simulink model "cusCommDemo_m"  (Simulink 6.0)
settings: Solver=FixedStepDiscrete  StartTime=0.0  StopTime=48  FixedStep=1  RelTol=1e-3
PostLoadFcn:
  | INC=uint8(1);LIMIT=uint8(16);RESET=uint8(0);K=int32(2);
libraries: mptlib x1
settings Model: CovMetricSettings=d  Creator=pszpak  LastModifiedBy=lzhang  ExtModeTrigMode=oneshot  ExtModeArmWhenConnect=off  ExtModeAutoUpdateStatusClock=off  BufferReuse=off  ProdHWDeviceType=Specified
settings DataIOCC: LimitDataPoints=off  SaveFormat=StructureWithTime  SaveOutput=off  SaveTime=off  SignalLoggingName=sigsOut
settings OptimizationCC: BlockReduction=off  InlineParams=on  BufferReuse=off  EnforceIntegerDowncast=off  LifeSpan=1
settings DebuggingCC: CheckExecutionContextPreStartOutputMsg=on  CheckExecutionContextRuntimeOutputMsg=on  SignalResolutionControl=TryResolveAll  SolverPrmCheckMsg=none  IntegerOverflowMsg=none
settings HardwareCC: ProdHWDeviceType=Specified
settings ModelReferenceCC: UpdateModelReferenceTargets=IfOutOfDate
settings RTWCC: SystemTargetFile=ert.tlc  TLCOptions=-aWarnNonSaturatedBlocks=0 -p0  TemplateMakefile=ert_default_tmf  GenerateReport=on  RTWVerbose=off  ProcessScript=ert_make_rtw_hook  IncludeHyperlinkInReport=on  LaunchReport=on
settings CodeAppCC: IgnoreCustomStorageClasses=off  PrefixModelToSubsysFcnNames=off  MangleLength=5  CustomCommentsFcn=custom_comments_example.m  EnableCustomComments=on
settings ERTTargetCC: TargetFcnLib=ansi_tfl_tmw.mat  GenFloatMathFcnCalls=ANSI_C  GenerateSampleERTMain=on  IncludeMdlTerminateFcn=off  SuppressErrorStatus=on  SupportContinuousTime=on  SupportNonInlinedSFcns=on  RootIOFormat=Individual Arguments  ERTSrcFileBannerTemplate=example_banner.tlc  ERTHdrFileBannerTemplate=example_banner.tlc  ERTDataSrcFileTemplate=example_banner.tlc  ERTDataHdrFileTemplate=example_banner.tlc  ERTCustomFileTemplate=example_file_process.tlc  InitialValueSource=DataObject
settings SFSimCC: SFSimApplyToAllLibs=on  SFSimBuildMode=Incremental

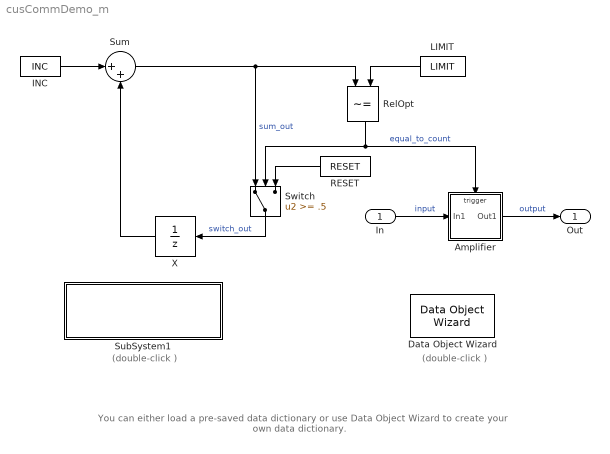
== system cusCommDemo_m ==
  note: (double-click )
  note: You can either load a pre-saved data dictionary or
      | use Data Object Wizard to create your own data dictionary.
  note: (double-click )
  In : Inport  DataType=int32  LatchInput=off
  Amplifier : Subsystem  TreatAsAtomicUnit=on  PropExecContextAcrossSSBoundary=on  RTWFileName=yyyyy
      settings: RTWSystemCode=Function
  Data Object Wizard : mptlib/Data Object Wizard  Description=DOW
  INC : Constant  Value=INC
  LIMIT : Constant  Orientation=left  Value=LIMIT
  RESET : Constant  Orientation=left  Value=RESET
  RelOpt : RelationalOperator  Orientation=down  Operator=~=  InputSameDT=on
  SubSystem1 : Subsystem  PropExecContextAcrossSSBoundary=on
      settings: OpenFcn=load cusCommDemo_ws
      mask Display: disp('Load pre-saved mat file\ncusCommDemo_ws');
  Sum : Sum  Inputs=|++  InputSameDT=on
  Switch : Switch  Orientation=down  Threshold=.5  SaturateOnIntegerOverflow=on  InputSameDT=on
  X : UnitDelay  Orientation=left  StateIdentifier=X
      settings: RTWStateStorageClass=ExportedGlobal
  Out : Outport
  wires:
  INC/1 -> Sum/1
  X/1 -> Sum/2
  Switch/1 -> X/1  "switch_out"
  Sum/1 -> Switch/1, RelOpt/1  "sum_out"
  LIMIT/1 -> RelOpt/2
  In/1 -> Amplifier/1(In1)  "input"
  RESET/1 -> Switch/3
  RelOpt/1 -> Switch/2, Amplifier/Trigger  "equal_to_count"
  Amplifier/1(Out1) -> Out/1  "output"

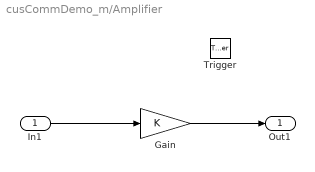
== system cusCommDemo_m/Amplifier ==
  In1 : Inport  LatchInput=off
  Trigger : TriggerPort
  Gain : Gain  Gain=K
  Out1 : Outport  InitialOutput=0
  wires:
  In1/1 -> Gain/1
  Gain/1 -> Out1/1

== system cusCommDemo_m/SubSystem1 ==
